simulink model "vct"  (Simulink 5.0)
settings: Solver=ode45  SolverMode=SingleTasking  StartTime=0.0  StopTime=.2  FixedStep=1e-4  MaxStep=.0001  RelTol=1e-3  AbsTol=1e-6
PreLoadFcn:
  | setup
values from neighbouring files (symbols this model uses):
  Kd = .0004    (= 0.0004)    [setup.m]    (also in vct_sys.m)
  Ki = .01    (= 0.01)    [setup.m]    (also in vct_sys.m)
  Kp = .025    (= 0.025)    [setup.m]    (also in vct_sys.m)
  ref = 18    [setup.m]    (also in vct_sys.m)
undefined symbols (not defined in the file or in its folder): get_linearcon_param, jitter, period, phase, vct_AR, vct_ICS
libraries: cmlib x4
settings Model: LastModifiedBy=ansgar  ExtModeTrigMode=oneshot  ExtModeArmWhenConnect=off  LimitDataPoints=off  BlockReductionOpt=off

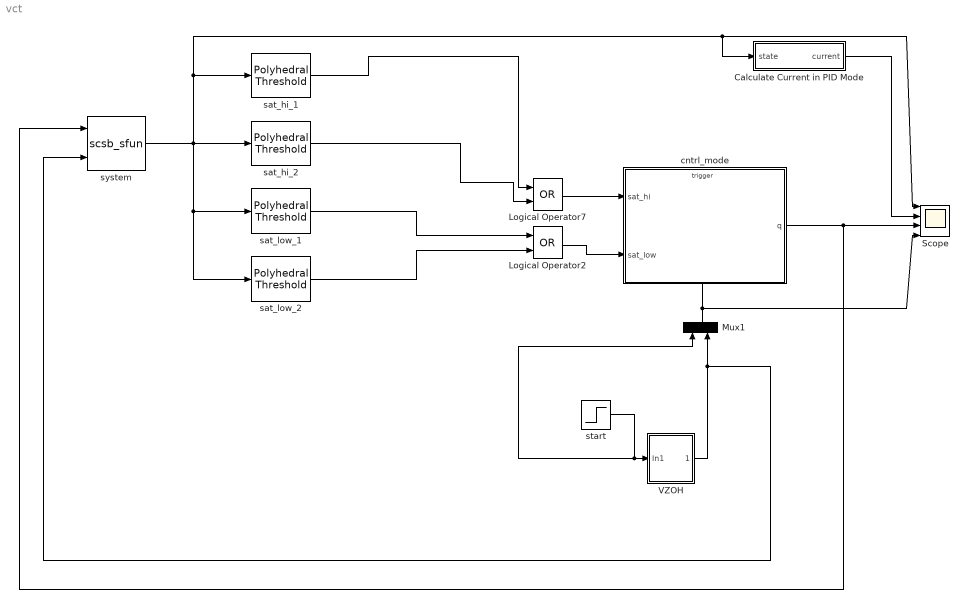
== system vct ==
  Calculate Current in PID Mode : Subsystem
  Logical Operator2 : Logic  Operator=OR
  Logical Operator7 : Logic  Operator=OR
  Mux1 : Mux  Orientation=up  Inputs=2
  Scope : Scope  NumInputPorts=4
      settings: TimeRange=0.12  YMin=-20~0.1~0~0  YMax=35~0.5~3~1  SaveName=test
  VZOH : Subsystem  AncestorBlock=cmlib/VZOH  mask(VariableZeroOrderHold){theta=phase, period=period, jitter=jitter}
      mask prompts: theta "Initial displacement"; period "Period of sampling time"; jitter "periodic Jitter"
      mask help: This block represents a Variable Zero-Order Hold Block. It enables the user to input a range for the initial displacement (theta), the period (delta) and the jitter(jitter). If the parameter is deterministic (e.g.: period = 5) it must be entered as an interval ( period = [5 5]). T. The block generates discrete-time impulse sequence in the output. For verification purposes, the user must include it in a stateflow diagram as "data input from simulink" and use it in conjunction with the guards to define the transition conditions. The input of this block is the "start" block, used to give the initial transition to the SFMB.
      mask Display: image(imread('clock1.jpg','jpeg'))
  cntrl_mode : Stateflow chart  TreatAsAtomicUnit=on
  sat_hi_1 : cmlib/Polyhedral Threshold  polyhedron=sat_hi_1
  sat_hi_2 : cmlib/Polyhedral Threshold  polyhedron=sat_hi_2
  sat_low_1 : cmlib/Polyhedral Threshold  polyhedron=sat_low_1
  sat_low_2 : cmlib/Polyhedral Threshold  polyhedron=sat_low_2
  start : Step  Time=.0001  SampleTime=0
  system : S-Function  AncestorBlock=cmlib/Switched Continuous System  FunctionName=scsb_sfun  Parameters=nx,nup,nz,nu,x0,swfunc,p0,use_reset,use_param,use_sd,get_linearcon_param(AR,'CI'),get_linearcon_param(AR,'dI')  mask(SwitchedContinuousSystem){nx=1, use_sd=on, nup=1, nz=2, use_reset=off, nu=1, x0=[0;0;0], swfunc=vct_sys, ICS=vct_ICS, AR=vct_AR, use_param=off, p0=[], PaCs=[]}
      mask prompts: nx "Number of Continuous States"; use_sd "Perform Sampled-Data Difference Equation Analysis"; nup "Number of Controller Outputs"; nz "Number of Discrete-Time Controller States"; use_reset "Show State Reset Port"; nu "Number of Integer Inputs from Stateflow Blocks"; x0 "Initial Conditions"; swfunc "Switching Function m-file"; ICS "Initial Continuous Set (@linearcon cell array from workspace)"; AR "Analysis Region (@linearcon from work space)"; use_param "Use Parameter Constraints"; p0 "Default Parameter"; PaCs "Parameter Constraints (@ linearcon from workspace)"
      mask help: This block represents a switched continuous dynamic system. The switching function is m-file function f(x,u) that outputs the continuous derivative xdot given continuous variable x and discrete (integer) input u. Initial continuous set and analysis region parameters are used for PIHA conversion purpose only. They do not affect the simulation result. They must be @linearcon objects imported from the main workspace in the MATLAB command window.
      mask init:
      | scsb_mask_handler(gcb)
      mask Display: plot(scsb_icon(1),scsb_icon(2))
  wires:
  Mux1/1 -> cntrl_mode/Trigger, Scope/4
  cntrl_mode/1(q) -> system/1, Scope/3
  start/1 -> Mux1/1, VZOH/1(In1)
  VZOH/1(Out1) -> Mux1/2, system/2
  system/1 -> sat_hi_2/1, sat_low_1/1, sat_low_2/1, sat_hi_1/1, Scope/1, Calculate Current in PID Mode/1(state)
  Calculate Current in PID Mode/1(current) -> Scope/2
  sat_hi_1/1 -> Logical Operator7/1
  sat_hi_2/1 -> Logical Operator7/2
  Logical Operator7/1 -> cntrl_mode/1(sat_hi)
  sat_low_1/1 -> Logical Operator2/1
  sat_low_2/1 -> Logical Operator2/2
  Logical Operator2/1 -> cntrl_mode/2(sat_low)

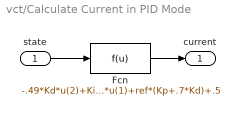
== system vct/Calculate Current in PID Mode ==
  state : Inport
  Fcn : Fcn  Expr=-.49*Kd*u(2)+Ki*u(3)-(Kp+.7*Kd)*u(1)+ref*(Kp+.7*Kd)+.5
  current : Outport
  wires:
  state/1 -> Fcn/1
  Fcn/1 -> current/1

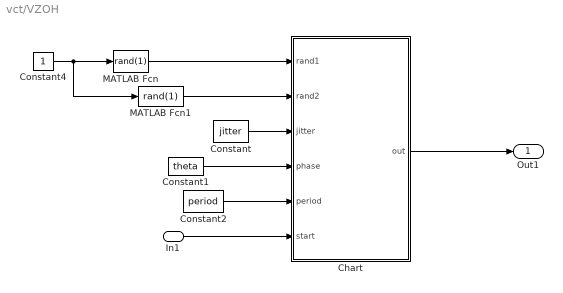
== system vct/VZOH ==
  In1 : Inport
  Chart : Stateflow chart
  Constant : Constant  Value=jitter
  Constant1 : Constant  Value=theta
  Constant2 : Constant  Value=period
  Constant4 : Constant
  MATLAB Fcn : MATLABFcn  MATLABFcn=rand(1)
  MATLAB Fcn1 : MATLABFcn  MATLABFcn=rand(1)
  Out1 : Outport
  wires:
  Chart/1(out) -> Out1/1
  Constant/1 -> Chart/3(jitter)
  Constant1/1 -> Chart/4(phase)
  Constant2/1 -> Chart/5(period)
  MATLAB Fcn1/1 -> Chart/2(rand2)
  MATLAB Fcn/1 -> Chart/1(rand1)
  In1/1 -> Chart/6(start)
  Constant4/1 -> MATLAB Fcn1/1, MATLAB Fcn/1

== stateflow chart cntrl_mode ==
  state pid
    entry: q = 3;
  state sat_low
    entry: q = 2;
  state sat_hi
    entry: q = 1;
  (default) -> sat_hi : start
  pid -> sat_hi : clock[(sat_hi==1)]
  sat_hi -> pid : clock[(~sat_hi==1)]
  sat_low -> pid : clock[(~sat_low==1)]
  pid -> sat_low : clock[(sat_low==1)]
  data: q output double; sat_hi input boolean; sat_low input boolean
  events: start input RISING_EDGE_EVENT; clock input RISING_EDGE_EVENT

== stateflow chart VZOH/Chart ==
  state calc/
    entry:
    out;
    sample_time=period[1]+rand1*(period[2]-period[1]);
    jitter_last=jitter_actual;
    jitter_actual=jitter[1]+rand2*(jitter[2]-jitter[1]);
    fire=sample_time-jitter_last+jitter_actual;
    time=t;
  state initial/
    entry:
    phase_actual=(phase[1]+rand1*(phase[2]-phase[1]));
    jitter_actual=jitter[1]+rand2*(jitter[2]-jitter[1]);
    fire=phase_actual+jitter_actual;
    time=t;
  state wait
  calc -> calc : [t-time>=fire]/out;
  initial -> calc : [t-time>=fire]/out;
  wait -> initial : [start>.5]
  (default) -> wait
  data: phase_actual local; jitter_actual local; fire local; time local; sample_time local; jitter_last local; rand1 input; rand2 input; jitter input size=2 =0; phase input size=2 =0; period input size=2 =0; start input
  events: out output EITHER_EDGE_EVENT
